simulink model "I_for_2_coils_linear_motion"  (R2021b)
settings: Solver=FixedStepAuto  StartTime=6.4e-3  StopTime=12.76e-3  FixedStep=50e-6  RelTol=1e-3
libraries: simulink x2
(part 1 of 2)
settings Model: Creator=teja  LastModifiedBy=teja

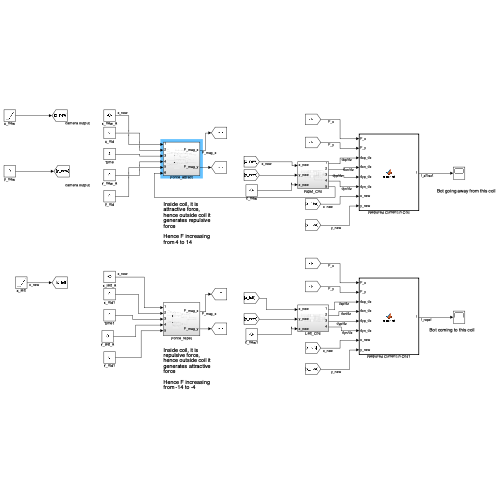
[thumbnail: Simulink's stored preview of the top-level diagram]
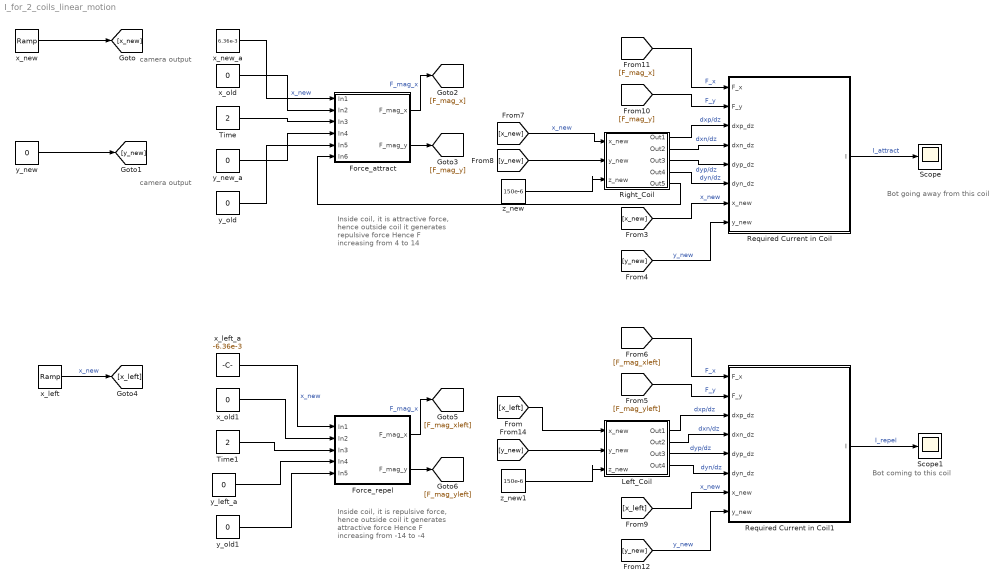
== system I_for_2_coils_linear_motion ==
  note: Bot going away from this coil
  note: Inside coil, it is attractive force, hence outside coil it generates repulsive force
      |
      | Hence F increasing from 4 to 14
  note: camera output
  note: camera output
  note: Inside coil, it is repulsive force, hence outside coil it generates attractive force
      |
      | Hence F increasing from -14 to -4
  note: Bot coming to this coil
  Force_attract : Subsystem
  Force_repel : Subsystem
  Left_Coil : Subsystem
  Required Current in Coil : MATLAB Function  TreatAsAtomicUnit=on
  Required Current in Coil1 : MATLAB Function  TreatAsAtomicUnit=on
  Right_Coil : Subsystem
  Scope : Scope
  Scope1 : Scope
  Time : Constant  Value=2
  Time1 : Constant  Value=2
  x_left : simulink/Sources/Ramp  slope=1  start=0  InitialOutput=-12.76e-3-6.4e-3
  x_left_a : Constant  Value=-6.36e-3
  x_new : simulink/Sources/Ramp  slope=1  start=0  InitialOutput=0
  x_new_a : Constant  Value=6.36e-3
  x_old : Constant  Value=0
  x_old1 : Constant  Value=0
  y_left_a : Constant  Value=0
  y_new : Constant  Value=0
  y_new_a : Constant  Value=0
  y_old : Constant  Value=0
  y_old1 : Constant  Value=0
  z_new : Constant  Value=150e-6
  z_new1 : Constant  Value=150e-6
  wires:
  x_old/1 -> Force_attract/2(In2)
  Time/1 -> Force_attract/3(In3)
  y_old/1 -> Force_attract/5(In5)
  x_new_a/1 -> Force_attract/1(In1)  "x_new"
  y_new/1 -> [y_new]
  y_new_a/1 -> Force_attract/4(In4)
  Force_attract/1(F_mag_x) -> [F_mag_x]  "F_mag_x"
  Force_attract/2(F_mag_y) -> [F_mag_y]
  [F_mag_x] -> Required Current in Coil/1(F_x)  "F_x"
  [F_mag_y] -> Required Current in Coil/2(F_y)  "F_y"
  [x_new] -> Right_Coil/1(x_new)  "x_new"
  [y_new] -> Right_Coil/2(y_new)
  z_new/1 -> Right_Coil/3(z_new)
  Right_Coil/1(Out1) -> Required Current in Coil/3(dxp_dz)  "dxp/dz"
  Right_Coil/2(Out2) -> Required Current in Coil/4(dxn_dz)  "dxn/dz"
  Right_Coil/3(Out3) -> Required Current in Coil/5(dyp_dz)  "dyp/dz"
  Right_Coil/4(Out4) -> Required Current in Coil/6(dyn_dz)  "dyn/dz"
  Required Current in Coil/1(I) -> Scope/1  "I_attract"
  [x_new] -> Required Current in Coil/7(x_new)  "x_new"
  [y_new] -> Required Current in Coil/8(y_new)  "y_new"
  [y_new] -> Required Current in Coil1/8(y_new)  "y_new"
  [x_left] -> Required Current in Coil1/7(x_new)  "x_new"
  Required Current in Coil1/1(I) -> Scope1/1  "I_repel"
  Left_Coil/4(Out4) -> Required Current in Coil1/6(dyn_dz)  "dyn/dz"
  Left_Coil/3(Out3) -> Required Current in Coil1/5(dyp_dz)  "dyp/dz"
  Left_Coil/2(Out2) -> Required Current in Coil1/4(dxn_dz)  "dxn/dz"
  Left_Coil/1(Out1) -> Required Current in Coil1/3(dxp_dz)  "dxp/dz"
  z_new1/1 -> Left_Coil/3(z_new)
  [y_new] -> Left_Coil/2(y_new)
  x_left/1 -> [x_left]  "x_new"
  [F_mag_yleft] -> Required Current in Coil1/2(F_y)  "F_y"
  [F_mag_xleft] -> Required Current in Coil1/1(F_x)  "F_x"
  x_new/1 -> [x_new]
  [x_left] -> Left_Coil/1(x_new)
  Force_repel/2(F_mag_y) -> [F_mag_yleft]
  Force_repel/1(F_mag_x) -> [F_mag_xleft]  "F_mag_x"
  y_left_a/1 -> Force_repel/4(In4)
  x_left_a/1 -> Force_repel/1(In1)  "x_new"
  y_old1/1 -> Force_repel/5(In5)
  Time1/1 -> Force_repel/3(In3)
  x_old1/1 -> Force_repel/2(In2)
  Right_Coil/5(Out5) -> Force_attract/6(In6)

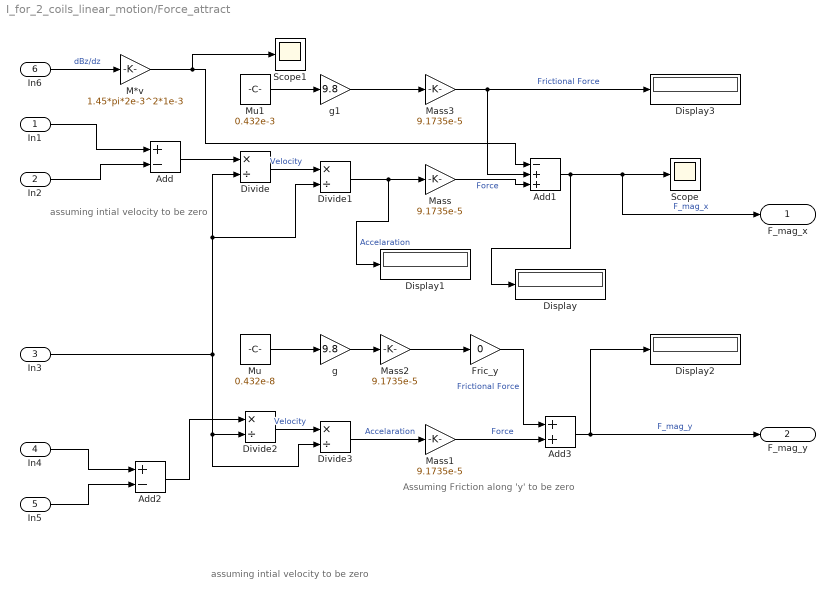
== system I_for_2_coils_linear_motion/Force_attract ==
  note: Assuming Friction along 'y' to be zero
  note: assuming intial velocity to be zero
  note: assuming intial velocity to be zero
  In1 : Inport
  In2 : Inport  Port=2
  In3 : Inport  Port=3
  In4 : Inport  Port=4
  In5 : Inport  Port=5
  In6 : Inport  Port=6
  Add : Sum  Inputs=+-
  Add1 : Sum  Inputs=-++
  Add2 : Sum  Inputs=+-
  Add3 : Sum
  Display{,1..3} (4 alike) : Display
  Divide{,1..3} (4 alike) : Product  Inputs=*/
  Fric_y : Gain  Gain=0
  M*v : Gain  Gain=1.45*pi*2e-3^2*1e-3
  Mass{,1..3} (4 alike) : Gain  Gain=9.1735e-5
  Mu : Constant  Value=0.432e-8
  Mu1 : Constant  Value=0.432e-3
  Scope : Scope
  Scope1 : Scope
  g : Gain  Gain=9.8
  g1 : Gain  Gain=9.8
  F_mag_x : Outport
  F_mag_y : Outport  Port=2
  wires:
  In4/1 -> Add2/1
  Add3/1 -> Display2/1, F_mag_y/1  "F_mag_y"
  In5/1 -> Add2/2
  Mass/1 -> Add1/3  "Force"
  Add2/1 -> Divide2/1
  Mass1/1 -> Add3/2  "Force"
  In1/1 -> Add/1
  Divide/1 -> Divide1/1  "Velocity"
  Add/1 -> Divide/1
  Divide2/1 -> Divide3/1  "Velocity"
  Divide3/1 -> Mass1/1  "Accelaration"
  Divide1/1 -> Display1/1, Mass/1  "Accelaration"
  In3/1 -> Divide/2, Divide1/2, Divide3/2, Divide2/2
  In2/1 -> Add/2
  Add1/1 -> Display/1, F_mag_x/1, Scope/1  "F_mag_x"
  Mu/1 -> g/1
  g/1 -> Mass2/1
  Mass3/1 -> Display3/1, Add1/2  "Frictional Force"
  g1/1 -> Mass3/1
  Mu1/1 -> g1/1
  Mass2/1 -> Fric_y/1
  Fric_y/1 -> Add3/1  "Frictional Force"
  In6/1 -> M*v/1  "dBz/dz"
  M*v/1 -> Scope1/1, Add1/1

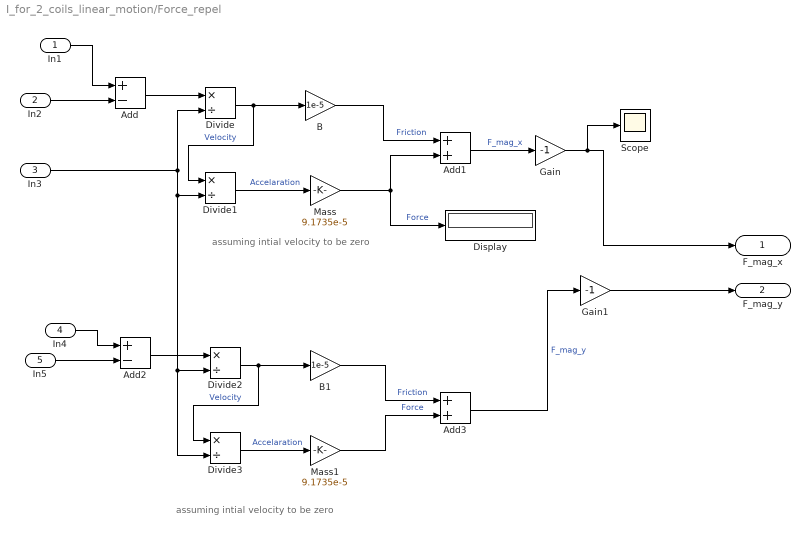
== system I_for_2_coils_linear_motion/Force_repel ==
  note: assuming intial velocity to be zero
  note: assuming intial velocity to be zero
  In1 : Inport
  In2 : Inport  Port=2
  In3 : Inport  Port=3
  In4 : Inport  Port=4
  In5 : Inport  Port=5
  Add : Sum  Inputs=+-
  Add1 : Sum
  Add2 : Sum  Inputs=+-
  Add3 : Sum
  B : Gain  Gain=1e-5
  B1 : Gain  Gain=1e-5
  Display : Display
  Divide{,1..3} (4 alike) : Product  Inputs=*/
  Gain : Gain  Gain=-1
  Gain1 : Gain  Gain=-1
  Mass : Gain  Gain=9.1735e-5
  Mass1 : Gain  Gain=9.1735e-5
  Scope : Scope
  F_mag_x : Outport
  F_mag_y : Outport  Port=2
  wires:
  Add1/1 -> Gain/1  "F_mag_x"
  In2/1 -> Add/2
  In3/1 -> Divide/2, Divide1/2, Divide2/2, Divide3/2
  Divide1/1 -> Mass/1  "Accelaration"
  Divide3/1 -> Mass1/1  "Accelaration"
  Divide2/1 -> Divide3/1, B1/1  "Velocity"
  Add/1 -> Divide/1
  Divide/1 -> B/1, Divide1/1  "Velocity"
  In1/1 -> Add/1
  B/1 -> Add1/1  "Friction"
  Mass1/1 -> Add3/2  "Force"
  B1/1 -> Add3/1  "Friction"
  Add2/1 -> Divide2/1
  Mass/1 -> Add1/2, Display/1  "Force"
  In5/1 -> Add2/2
  Add3/1 -> Gain1/1  "F_mag_y"
  In4/1 -> Add2/1
  Gain/1 -> F_mag_x/1, Scope/1
  Gain1/1 -> F_mag_y/1

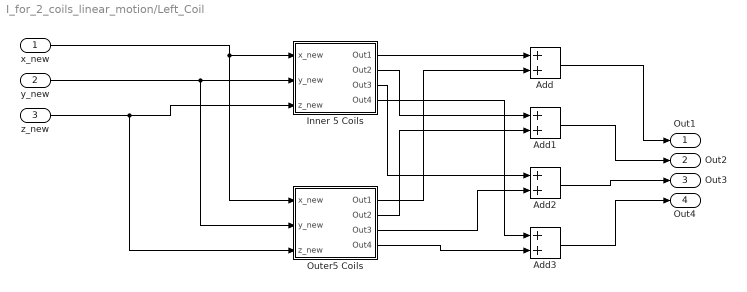
== system I_for_2_coils_linear_motion/Left_Coil ==
  x_new : Inport
  y_new : Inport  Port=2
  z_new : Inport  Port=3
  Add{,1..3} (4 alike) : Sum
  Inner 5 Coils : Subsystem
  Outer5 Coils : Subsystem
  Out1 : Outport
  Out2 : Outport  Port=2
  Out3 : Outport  Port=3
  Out4 : Outport  Port=4
  wires:
  z_new/1 -> Inner 5 Coils/3(z_new), Outer5 Coils/3(z_new)
  Outer5 Coils/4(Out4) -> Add3/2
  Outer5 Coils/1(Out1) -> Add/2
  y_new/1 -> Inner 5 Coils/2(y_new), Outer5 Coils/2(y_new)
  Inner 5 Coils/1(Out1) -> Add/1
  Inner 5 Coils/2(Out2) -> Add1/1
  x_new/1 -> Inner 5 Coils/1(x_new), Outer5 Coils/1(x_new)
  Inner 5 Coils/4(Out4) -> Add3/1
  Add3/1 -> Out4/1
  Inner 5 Coils/3(Out3) -> Add2/1
  Add/1 -> Out1/1
  Outer5 Coils/3(Out3) -> Add2/2
  Outer5 Coils/2(Out2) -> Add1/2
  Add1/1 -> Out2/1
  Add2/1 -> Out3/1

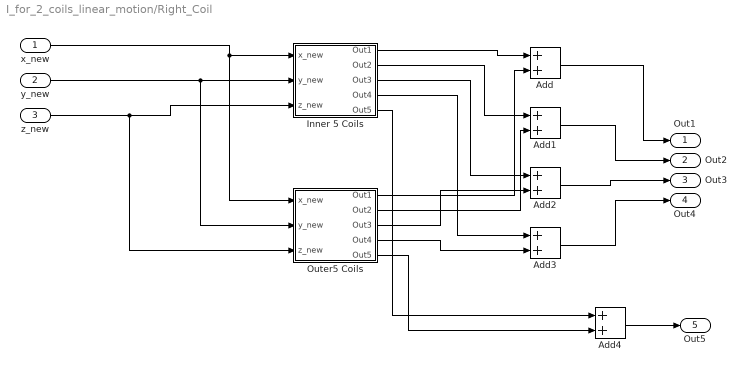
== system I_for_2_coils_linear_motion/Right_Coil ==
  x_new : Inport
  y_new : Inport  Port=2
  z_new : Inport  Port=3
  Add{,1..4} (5 alike) : Sum
  Inner 5 Coils : Subsystem
  Outer5 Coils : Subsystem
  Out1 : Outport
  Out2 : Outport  Port=2
  Out3 : Outport  Port=3
  Out4 : Outport  Port=4
  Out5 : Outport  Port=5
  wires:
  Add2/1 -> Out3/1
  Add1/1 -> Out2/1
  Outer5 Coils/2(Out2) -> Add1/2
  Outer5 Coils/3(Out3) -> Add2/2
  Add/1 -> Out1/1
  Inner 5 Coils/3(Out3) -> Add2/1
  Add3/1 -> Out4/1
  Inner 5 Coils/4(Out4) -> Add3/1
  x_new/1 -> Outer5 Coils/1(x_new), Inner 5 Coils/1(x_new)
  Inner 5 Coils/2(Out2) -> Add1/1
  Inner 5 Coils/1(Out1) -> Add/1
  y_new/1 -> Outer5 Coils/2(y_new), Inner 5 Coils/2(y_new)
  Outer5 Coils/1(Out1) -> Add/2
  Outer5 Coils/4(Out4) -> Add3/2
  z_new/1 -> Outer5 Coils/3(z_new), Inner 5 Coils/3(z_new)
  Outer5 Coils/5(Out5) -> Add4/2
  Inner 5 Coils/5(Out5) -> Add4/1
  Add4/1 -> Out5/1

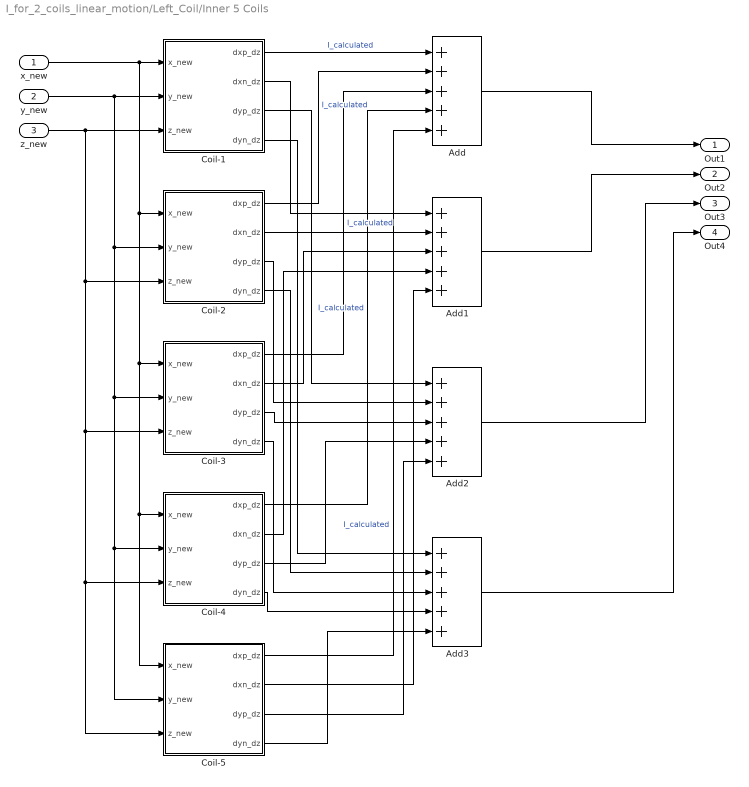
== system I_for_2_coils_linear_motion/Left_Coil/Inner 5 Coils ==
  x_new : Inport
  y_new : Inport  Port=2
  z_new : Inport  Port=3
  Add{,1..3} (4 alike) : Sum  Inputs=+++++
  Coil-1 : MATLAB Function  TreatAsAtomicUnit=on
  Coil-2 : MATLAB Function  TreatAsAtomicUnit=on
  Coil-3 : MATLAB Function  TreatAsAtomicUnit=on
  Coil-4 : MATLAB Function  TreatAsAtomicUnit=on
  Coil-5 : MATLAB Function  TreatAsAtomicUnit=on
  Out1 : Outport
  Out2 : Outport  Port=2
  Out3 : Outport  Port=3
  Out4 : Outport  Port=4
  wires:
  Coil-5/2(dxn_dz) -> Add1/5
  Coil-3/3(dyp_dz) -> Add2/3
  Coil-3/2(dxn_dz) -> Add1/3
  Coil-4/2(dxn_dz) -> Add1/4
  Coil-5/4(dyn_dz) -> Add3/5
  Coil-4/3(dyp_dz) -> Add2/4
  Coil-5/3(dyp_dz) -> Add2/5
  Coil-2/3(dyp_dz) -> Add2/2
  Coil-1/1(dxp_dz) -> Add/1  "I_calculated"
  x_new/1 -> Coil-1/1(x_new), Coil-2/1(x_new), Coil-3/1(x_new), Coil-4/1(x_new), Coil-5/1(x_new)
  Coil-5/1(dxp_dz) -> Add/5  "I_calculated"
  y_new/1 -> Coil-1/2(y_new), Coil-2/2(y_new), Coil-3/2(y_new), Coil-4/2(y_new), Coil-5/2(y_new)
  Coil-1/4(dyn_dz) -> Add3/1
  Coil-4/4(dyn_dz) -> Add3/4
  Coil-1/2(dxn_dz) -> Add1/1
  Coil-1/3(dyp_dz) -> Add2/1
  Coil-2/1(dxp_dz) -> Add/2  "I_calculated"
  Add/1 -> Out1/1
  Coil-4/1(dxp_dz) -> Add/4  "I_calculated"
  z_new/1 -> Coil-2/3(z_new), Coil-5/3(z_new), Coil-4/3(z_new), Coil-3/3(z_new), Coil-1/3(z_new)
  Coil-3/4(dyn_dz) -> Add3/3
  Coil-3/1(dxp_dz) -> Add/3  "I_calculated"
  Add3/1 -> Out4/1
  Coil-2/4(dyn_dz) -> Add3/2
  Coil-2/2(dxn_dz) -> Add1/2
  Add1/1 -> Out2/1
  Add2/1 -> Out3/1

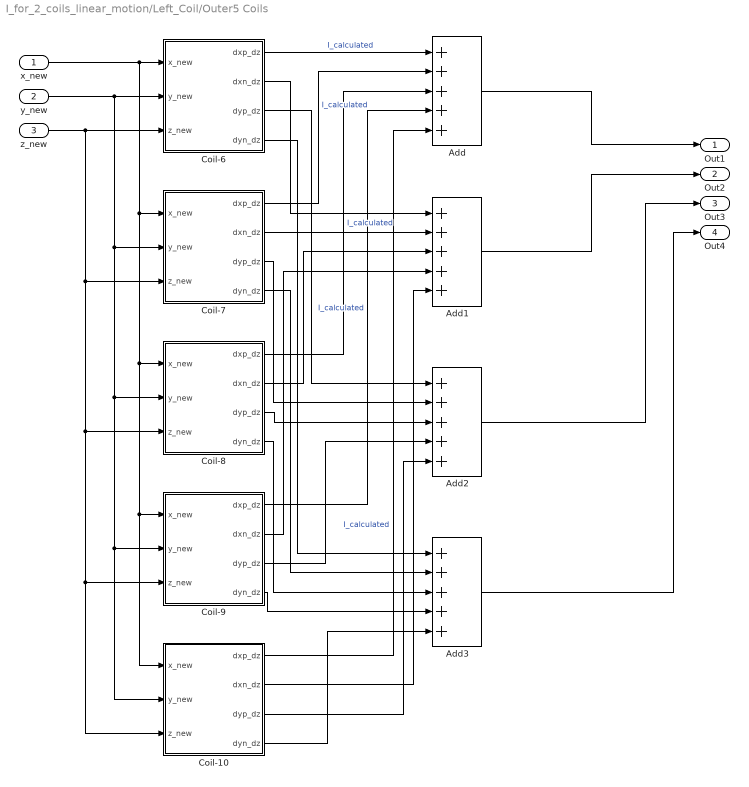
== system I_for_2_coils_linear_motion/Left_Coil/Outer5 Coils ==
  x_new : Inport
  y_new : Inport  Port=2
  z_new : Inport  Port=3
  Add{,1..3} (4 alike) : Sum  Inputs=+++++
  Coil-10 : MATLAB Function  TreatAsAtomicUnit=on
  Coil-6 : MATLAB Function  TreatAsAtomicUnit=on
  Coil-7 : MATLAB Function  TreatAsAtomicUnit=on
  Coil-8 : MATLAB Function  TreatAsAtomicUnit=on
  Coil-9 : MATLAB Function  TreatAsAtomicUnit=on
  Out1 : Outport
  Out2 : Outport  Port=2
  Out3 : Outport  Port=3
  Out4 : Outport  Port=4
  wires:
  Add2/1 -> Out3/1
  Add1/1 -> Out2/1
  Coil-7/2(dxn_dz) -> Add1/2
  Coil-7/4(dyn_dz) -> Add3/2
  Add3/1 -> Out4/1
  Coil-8/1(dxp_dz) -> Add/3  "I_calculated"
  Coil-8/4(dyn_dz) -> Add3/3
  z_new/1 -> Coil-6/3(z_new), Coil-8/3(z_new), Coil-10/3(z_new), Coil-9/3(z_new), Coil-7/3(z_new)
  Coil-9/1(dxp_dz) -> Add/4  "I_calculated"
  Add/1 -> Out1/1
  Coil-7/1(dxp_dz) -> Add/2  "I_calculated"
  Coil-6/3(dyp_dz) -> Add2/1
  Coil-6/2(dxn_dz) -> Add1/1
  Coil-9/4(dyn_dz) -> Add3/4
  Coil-6/4(dyn_dz) -> Add3/1
  y_new/1 -> Coil-10/2(y_new), Coil-9/2(y_new), Coil-8/2(y_new), Coil-7/2(y_new), Coil-6/2(y_new)
  Coil-10/1(dxp_dz) -> Add/5  "I_calculated"
  x_new/1 -> Coil-10/1(x_new), Coil-9/1(x_new), Coil-8/1(x_new), Coil-7/1(x_new), Coil-6/1(x_new)
  Coil-6/1(dxp_dz) -> Add/1  "I_calculated"
  Coil-7/3(dyp_dz) -> Add2/2
  Coil-10/3(dyp_dz) -> Add2/5
  Coil-9/3(dyp_dz) -> Add2/4
  Coil-10/4(dyn_dz) -> Add3/5
  Coil-9/2(dxn_dz) -> Add1/4
  Coil-8/2(dxn_dz) -> Add1/3
  Coil-8/3(dyp_dz) -> Add2/3
  Coil-10/2(dxn_dz) -> Add1/5

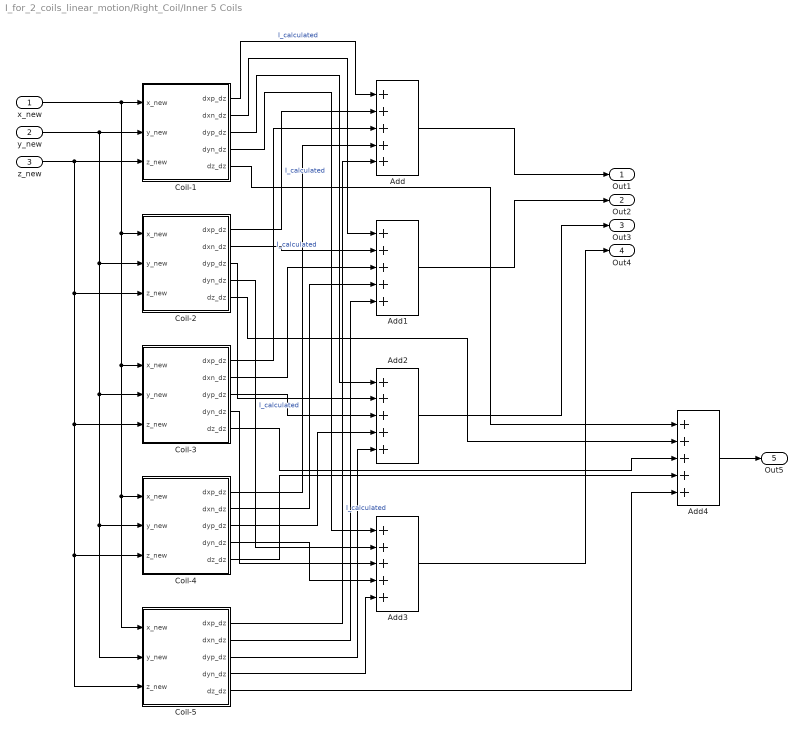
== system I_for_2_coils_linear_motion/Right_Coil/Inner 5 Coils ==
  x_new : Inport
  y_new : Inport  Port=2
  z_new : Inport  Port=3
  Add{,1..4} (5 alike) : Sum  Inputs=+++++
  Coil-1 : MATLAB Function  TreatAsAtomicUnit=on
  Coil-2 : MATLAB Function  TreatAsAtomicUnit=on
  Coil-3 : MATLAB Function  TreatAsAtomicUnit=on
  Coil-4 : MATLAB Function  TreatAsAtomicUnit=on
  Coil-5 : MATLAB Function  TreatAsAtomicUnit=on
  Out1 : Outport
  Out2 : Outport  Port=2
  Out3 : Outport  Port=3
  Out4 : Outport  Port=4
  Out5 : Outport  Port=5
  wires:
  Add2/1 -> Out3/1
  Add1/1 -> Out2/1
  Coil-2/2(dxn_dz) -> Add1/2
  Coil-2/4(dyn_dz) -> Add3/2
  Add3/1 -> Out4/1
  Coil-3/1(dxp_dz) -> Add/3  "I_calculated"
  Coil-3/4(dyn_dz) -> Add3/3
  z_new/1 -> Coil-1/3(z_new), Coil-3/3(z_new), Coil-4/3(z_new), Coil-5/3(z_new), Coil-2/3(z_new)
  Coil-4/1(dxp_dz) -> Add/4  "I_calculated"
  Add/1 -> Out1/1
  Coil-2/1(dxp_dz) -> Add/2  "I_calculated"
  Coil-1/3(dyp_dz) -> Add2/1
  Coil-1/2(dxn_dz) -> Add1/1
  Coil-4/4(dyn_dz) -> Add3/4
  Coil-1/4(dyn_dz) -> Add3/1
  y_new/1 -> Coil-5/2(y_new), Coil-4/2(y_new), Coil-3/2(y_new), Coil-2/2(y_new), Coil-1/2(y_new)
  Coil-5/1(dxp_dz) -> Add/5  "I_calculated"
  x_new/1 -> Coil-5/1(x_new), Coil-4/1(x_new), Coil-3/1(x_new), Coil-2/1(x_new), Coil-1/1(x_new)
  Coil-1/1(dxp_dz) -> Add/1  "I_calculated"
  Coil-2/3(dyp_dz) -> Add2/2
  Coil-5/3(dyp_dz) -> Add2/5
  Coil-4/3(dyp_dz) -> Add2/4
  Coil-5/4(dyn_dz) -> Add3/5
  Coil-4/2(dxn_dz) -> Add1/4
  Coil-3/2(dxn_dz) -> Add1/3
  Coil-3/3(dyp_dz) -> Add2/3
  Coil-5/2(dxn_dz) -> Add1/5
  Coil-1/5(dz_dz) -> Add4/1
  Coil-2/5(dz_dz) -> Add4/2
  Coil-3/5(dz_dz) -> Add4/3
  Coil-4/5(dz_dz) -> Add4/4
  Coil-5/5(dz_dz) -> Add4/5
  Add4/1 -> Out5/1

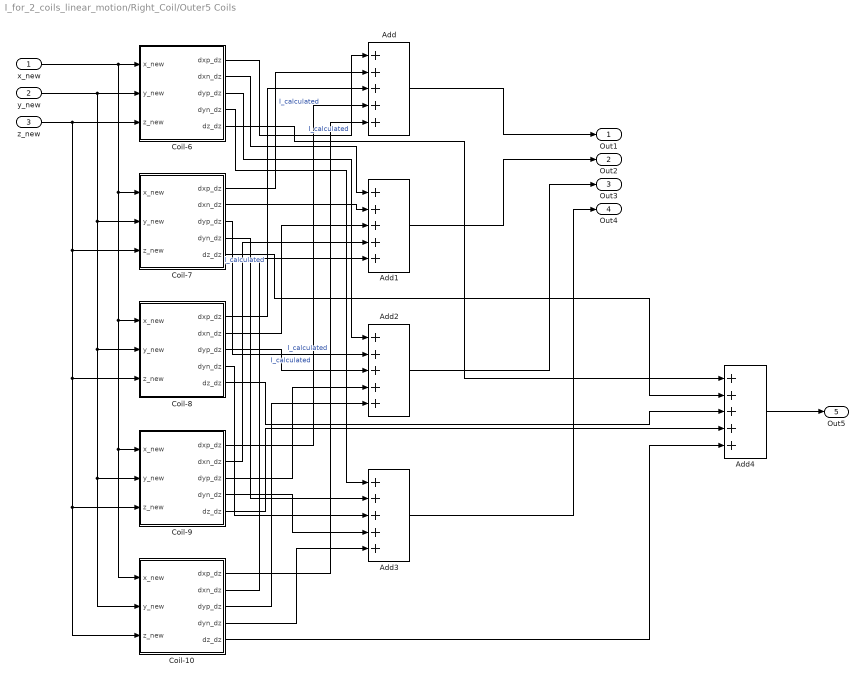
== system I_for_2_coils_linear_motion/Right_Coil/Outer5 Coils ==
  x_new : Inport
  y_new : Inport  Port=2
  z_new : Inport  Port=3
  Add{,1..4} (5 alike) : Sum  Inputs=+++++
  Coil-10 : MATLAB Function  TreatAsAtomicUnit=on
  Coil-6 : MATLAB Function  TreatAsAtomicUnit=on
  Coil-7 : MATLAB Function  TreatAsAtomicUnit=on
  Coil-8 : MATLAB Function  TreatAsAtomicUnit=on
  Coil-9 : MATLAB Function  TreatAsAtomicUnit=on
  Out1 : Outport
  Out2 : Outport  Port=2
  Out3 : Outport  Port=3
  Out4 : Outport  Port=4
  Out5 : Outport  Port=5
  wires:
  Coil-10/2(dxn_dz) -> Add1/5
  Coil-8/3(dyp_dz) -> Add2/3
  Coil-8/2(dxn_dz) -> Add1/3
  Coil-9/2(dxn_dz) -> Add1/4
  Coil-10/4(dyn_dz) -> Add3/5
  Coil-9/3(dyp_dz) -> Add2/4
  Coil-10/3(dyp_dz) -> Add2/5
  Coil-7/3(dyp_dz) -> Add2/2
  Coil-6/1(dxp_dz) -> Add/1  "I_calculated"
  x_new/1 -> Coil-6/1(x_new), Coil-7/1(x_new), Coil-8/1(x_new), Coil-9/1(x_new), Coil-10/1(x_new)
  Coil-10/1(dxp_dz) -> Add/5  "I_calculated"
  y_new/1 -> Coil-6/2(y_new), Coil-7/2(y_new), Coil-8/2(y_new), Coil-9/2(y_new), Coil-10/2(y_new)
  Coil-6/4(dyn_dz) -> Add3/1
  Coil-9/4(dyn_dz) -> Add3/4
  Coil-6/2(dxn_dz) -> Add1/1
  Coil-6/3(dyp_dz) -> Add2/1
  Coil-7/1(dxp_dz) -> Add/2  "I_calculated"
  Add/1 -> Out1/1
  Coil-9/1(dxp_dz) -> Add/4  "I_calculated"
  z_new/1 -> Coil-7/3(z_new), Coil-9/3(z_new), Coil-10/3(z_new), Coil-8/3(z_new), Coil-6/3(z_new)
  Coil-8/4(dyn_dz) -> Add3/3
  Coil-8/1(dxp_dz) -> Add/3  "I_calculated"
  Add3/1 -> Out4/1
  Coil-7/4(dyn_dz) -> Add3/2
  Coil-7/2(dxn_dz) -> Add1/2
  Add1/1 -> Out2/1
  Add2/1 -> Out3/1
  Coil-6/5(dz_dz) -> Add4/1
  Coil-7/5(dz_dz) -> Add4/2
  Coil-8/5(dz_dz) -> Add4/3
  Coil-9/5(dz_dz) -> Add4/4
  Coil-10/5(dz_dz) -> Add4/5
  Add4/1 -> Out5/1

== matlab function I_for_2_coils_linear_motion/Required Current in Coil ==
  data: F_x input; F_y input; I output; dxp_dz input; dxn_dz input; dyp_dz input; dyn_dz input; x_new input; y_new input
function  I = current(F_x, F_y,dxp_dz, dxn_dz, dyp_dz, dyn_dz, x_new, y_new)
radius = 3e-3;%m
height = 1e-3;%m
Magentization = 1.45; %T
m0 = 4*pi*10e-7;
vol_cy = pi*radius^2*height; % If Object is Cylinder, vol in m^3
if F_y == 0 && x_new ~= 0
        I = (F_x/ (dxp_dz + dxn_dz))* m0/ (vol_cy * Magentization);
    elseif F_x == 0 && y_new ~= 0
        I = (F_y / (dyp_dz + dyn_dz))* m0/ (vol_cy * Magentization);
    elseif F_x== 0 && F_y == 0 
        I = 0;
    else
        I = (F_x/ (dxp_dz + dxn_dz)+  F_y / (dyp_dz + dyn_dz))* m0/ (vol_cy * Magentization);
end
end

== matlab function I_for_2_coils_linear_motion/Right_Coil/Outer5 Coils/Coil-6 ==
  data: dxp_dz output; x_new input; y_new input; z_new input; dxn_dz output; dyp_dz output; dyn_dz output; dz_dz output
function  [dxp_dz, dxn_dz, dyp_dz, dyn_dz, dz_dz] = current(x_new, y_new, z_new)

g = 420e-6;     %Coil spacing
m0 = 4*pi*1e-7;
radius = 3e-3;%m
height = 1e-3;%m
Magentization = 1.45; %T
vol_cy = pi*radius^2*height; % If Object is Cylinder, vol in m^3
% vol_sp = (4/3)*(pi * radius^3); % If Object is Sphere, vol in m^3

k = 0.4e-3; %additional length added to wires, to get concentric coil
%--------%--------%--------%--------%--------%--------%--------%----------
% Line along y - axis
%-%--------%--------%--------%--------%--------%--------%--------%--------
yp1_1 = -0.6e-3 - 5*k;
yp2_1 = 0.6e-3 + 5*k;
yn1_1 = -0.8e-3 - 5*k;
yn2_1 = 0.8e-3 + 5*k;
a_xp_1 = 6*g;  
a_xn_1 = -6*g;

k_yp_1 = 1/(4*pi*((a_xp_1-x_new)^2+z_new^2));
k_1yp_1 = (yp2_1-y_new)/((yp2_1-y_new)^2+(a_xp_1-x_new)^2+z_new^2)^0.5;
k_2yp_1 = (yp1_1-y_new)/((yp1_1-y_new)^2+(a_xp_1-x_new)^2+z_new^2)^0.5;

k_1yp_3 = (yp2_1-y_new)/((yp2_1-y_new)^2+(a_xp_1-x_new)^2+z_new^2)^1.5;
k_2yp_3 = (yp1_1-y_new)/((yp1_1-y_new)^2+(a_xp_1-x_new)^2+z_new^2)^1.5;

k_yn_1 = 1/(4*pi*((a_xn_1-x_new)^2+z_new^2));
k_1yn_1 = (yn2_1-y_new)/((yn2_1-y_new)^2+(a_xn_1-x_new)^2+z_new^2)^0.5;
k_2yn_1 = (yn1_1-y_new)/((yn1_1-y_new)^2+(a_xn_1-x_new)^2+z_new^2)^0.5;

k_1yn_3 = (yn2_1-y_new)/((yn2_1-y_new)^2+(a_xn_1-x_new)^2+z_new^2)^1.5;
k_2yn_3 = (yn1_1-y_new)/((yn1_1-y_new)^2+(a_xn_1-x_new)^2+z_new^2)^1.5;


hyp_z_1 = (k_yp_1) *m0;
hyp_z1_1 = (k_1yp_1 - k_2yp_1)*(-1);
hyp_z2_1 = (k_yp_1*(k_1yp_1 - k_2yp_1)*(z_new^2))*4*pi*2;
hyp_z3_1 = (k_1yp_3 - k_2yp_3)*(z_new^2);
dxp_dz = hyp_z_1*(hyp_z1_1 + hyp_z2_1 + hyp_z3_1);


hyn_z_1 = (k_yn_1)* m0*(-1);
hyn_z1_1 = (k_1yn_1 - k_2yn_1)*(-1);
hyn_z2_1 = (k_yn_1*(k_1yn_1 - k_2yn_1)*(z_new^2))*4*pi*2;
hyn_z3_1 = (k_1yn_3 - k_2yn_3)*(z_new^2);
dxn_dz = hyn_z_1*(hyn_z1_1 + hyn_z2_1 + hyn_z3_1);

%--------%--------%--------%--------%--------%--------%--------%----------
% Line along x - axis
%-%--------%--------%--------%--------%a--------%--------%--------%--------
xp1_1 = -0.8e-3 - 5*k;
xp2_1 = 0.8e-3 + 5*k;
xn1_1 = -1e-3 - 5*k;
xn2_1 = 1e-3 + 5*k;
a_yp_1 = 2.675;          %Distance of coil from (0,0)
a_yn_1 = -2.675;

k_xp_1 = 1/(4*pi*((a_yp_1-y_new)^2+z_new^2));
k_1xp_1 = (xp2_1-x_new)/((xp2_1-x_new)^2+(a_yp_1-y_new)^2+z_new^2)^0.5;
k_2xp_1 = (xp1_1-x_new)/((xp1_1-x_new)^2+(a_yp_1-y_new)^2+z_new^2)^0.5;

k_xn_1 = 1/(4*pi*((a_yn_1-y_new)^2+z_new^2));
k_1xn_1 = (xn2_1-x_new)/((xn2_1-x_new)^2+(a_yn_1-y_new)^2+z_new^2)^0.5;
k_2xn_1 = (xn1_1-x_new)/((xn1_1-x_new)^2+(a_yn_1-y_new)^2+z_new^2)^0.5;

k_1xp_3 = (xp2_1-x_new)/((xp2_1-x_new)^2+(a_yp_1-y_new)^2+z_new^2)^1.5;
k_2xp_3 = (xp1_1-x_new)/((xp1_1-x_new)^2+(a_yp_1-y_new)^2+z_new^2)^1.5;

k_1xn_3 = (xn2_1-x_new)/((xn2_1-x_new)^2+(a_yn_1-y_new)^2+z_new^2)^1.5;
k_2xn_3 = (xn1_1-x_new)/((xn1_1-x_new)^2+(a_yn_1-y_new)^2+z_new^2)^1.5;


hxp_z_1 = (k_xp_1)*m0;
hxp_z1_1 = (k_1xp_1 - k_2xp_1)*(-1);
hxp_z2_1 = (k_xp_1*(k_1xp_1 - k_2xp_1)*(z_new^2))*4*pi*2;
hxp_z3_1 = (k_1xp_3 - k_2xp_3)*(z_new^2);
dyp_dz = hxp_z_1*(hxp_z1_1 + hxp_z2_1 + hxp_z3_1);


hxn_z_1 = (k_xn_1)*m0*(-1);
hxn_z1_1 = (k_1xn_1 - k_2xn_1)*(-1);
hxn_z2_1 = (k_xn_1*(k_1xn_1 - k_2xn_1)*(z_new^2))*4*pi*2;
hxn_z3_1 = (k_1xn_3 - k_2xn_3)*(z_new^2);
dyn_dz = hxn_z_1*(hxn_z1_1 + hxn_z2_1 + hxn_z3_1);

hzp_z_1 = (k_yp_1) *m0 * ((a_yp_1-y_new)+(a_xp_1-x_new)) * z_new ;
hzp_z1_1 = (k_1yp_1 - k_2yp_1 + k_1xp_1 - k_2xp_1)*(-2);
hzp_z3_1 = (k_1yp_3 - k_2yp_3 + k_1xp_3 - k_2xp_3);
dzp_dz = hzp_z_1*(hzp_z1_1 + hzp_z3_1);

hzn_z_1 = (k_yp_1) *m0 *(-1) * ((a_yn_1-y_new)+(a_xn_1-x_new)) * z_new;
hzn_z1_1 =(k_1yn_1 - k_2yn_1 + k_1xn_1 - k_2xn_1)*(-2);
hzn_z3_1 = (k_1yn_3 - k_2yn_3 + k_1xn_3 - k_2xn_3);
dzn_dz = hzn_z_1*(hzn_z1_1 + hzn_z3_1);

dz_dz = dzp_dz + dzn_dz;

end

== matlab function I_for_2_coils_linear_motion/Right_Coil/Outer5 Coils/Coil-7 ==
  data: dxp_dz output; x_new input; y_new input; z_new input; dxn_dz output; dyp_dz output; dyn_dz output; dz_dz output
function  [dxp_dz, dxn_dz, dyp_dz, dyn_dz, dz_dz] = current(x_new, y_new, z_new)

g = 417.14e-6;     %Coil spacing
m0 = 4*pi*1e-7;
radius = 3e-3;%m
height = 1e-3;%m
Magentization = 1.45; %T
vol_cy = pi*radius^2*height; % If Object is Cylinder, vol in m^3
% vol_sp = (4/3)*(pi * radius^3); % If Object is Sphere, vol in m^3

k = 0.4e-3; %additional length added to wires, to get concentric coil
%--------%--------%--------%--------%--------%--------%--------%----------
% Line along y - axis
%-%--------%--------%--------%--------%--------%--------%--------%--------
yp1_1 = -0.6e-3 - 6*k;
yp2_1 = 0.6e-3 + 6*k;
yn1_1 = -0.8e-3 - 6*k;
yn2_1 = 0.8e-3 + 6*k;
a_xp_1 = 7*g;  
a_xn_1 = -7*g;

k_yp_1 = 1/(4*pi*((a_xp_1-x_new)^2+z_new^2));
k_1yp_1 = (yp2_1-y_new)/((yp2_1-y_new)^2+(a_xp_1-x_new)^2+z_new^2)^0.5;
k_2yp_1 = (yp1_1-y_new)/((yp1_1-y_new)^2+(a_xp_1-x_new)^2+z_new^2)^0.5;

k_1yp_3 = (yp2_1-y_new)/((yp2_1-y_new)^2+(a_xp_1-x_new)^2+z_new^2)^1.5;
k_2yp_3 = (yp1_1-y_new)/((yp1_1-y_new)^2+(a_xp_1-x_new)^2+z_new^2)^1.5;

k_yn_1 = 1/(4*pi*((a_xn_1-x_new)^2+z_new^2));
k_1yn_1 = (yn2_1-y_new)/((yn2_1-y_new)^2+(a_xn_1-x_new)^2+z_new^2)^0.5;
k_2yn_1 = (yn1_1-y_new)/((yn1_1-y_new)^2+(a_xn_1-x_new)^2+z_new^2)^0.5;

k_1yn_3 = (yn2_1-y_new)/((yn2_1-y_new)^2+(a_xn_1-x_new)^2+z_new^2)^1.5;
k_2yn_3 = (yn1_1-y_new)/((yn1_1-y_new)^2+(a_xn_1-x_new)^2+z_new^2)^1.5;


hyp_z_1 = (k_yp_1) *m0;
hyp_z1_1 = (k_1yp_1 - k_2yp_1)*(-1);
hyp_z2_1 = (k_yp_1*(k_1yp_1 - k_2yp_1)*(z_new^2))*4*pi*2;
hyp_z3_1 = (k_1yp_3 - k_2yp_3)*(z_new^2);
dxp_dz = hyp_z_1*(hyp_z1_1 + hyp_z2_1 + hyp_z3_1);


hyn_z_1 = (k_yn_1)* m0*(-1);
hyn_z1_1 = (k_1yn_1 - k_2yn_1)*(-1);
hyn_z2_1 = (k_yn_1*(k_1yn_1 - k_2yn_1)*(z_new^2))*4*pi*2;
hyn_z3_1 = (k_1yn_3 - k_2yn_3)*(z_new^2);
dxn_dz = hyn_z_1*(hyn_z1_1 + hyn_z2_1 + hyn_z3_1);

%--------%--------%--------%--------%--------%--------%--------%----------
% Line along x - axis
%-%--------%--------%--------%--------%a--------%--------%--------%--------
xp1_1 = -0.8e-3 - 6*k;
xp2_1 = 0.8e-3 + 6*k;
xn1_1 = -1e-3 - 6*k;
xn2_1 = 1e-3 + 6*k;
a_yp_1 = 3.075;          %Distance of coil from (0,0)
a_yn_1 = -3.075;

k_xp_1 = 1/(4*pi*((a_yp_1-y_new)^2+z_new^2));
k_1xp_1 = (xp2_1-x_new)/((xp2_1-x_new)^2+(a_yp_1-y_new)^2+z_new^2)^0.5;
k_2xp_1 = (xp1_1-x_new)/((xp1_1-x_new)^2+(a_yp_1-y_new)^2+z_new^2)^0.5;

k_xn_1 = 1/(4*pi*((a_yn_1-y_new)^2+z_new^2));
k_1xn_1 = (xn2_1-x_new)/((xn2_1-x_new)^2+(a_yn_1-y_new)^2+z_new^2)^0.5;
k_2xn_1 = (xn1_1-x_new)/((xn1_1-x_new)^2+(a_yn_1-y_new)^2+z_new^2)^0.5;

k_1xp_3 = (xp2_1-x_new)/((xp2_1-x_new)^2+(a_yp_1-y_new)^2+z_new^2)^1.5;
k_2xp_3 = (xp1_1-x_new)/((xp1_1-x_new)^2+(a_yp_1-y_new)^2+z_new^2)^1.5;

k_1xn_3 = (xn2_1-x_new)/((xn2_1-x_new)^2+(a_yn_1-y_new)^2+z_new^2)^1.5;
k_2xn_3 = (xn1_1-x_new)/((xn1_1-x_new)^2+(a_yn_1-y_new)^2+z_new^2)^1.5;


hxp_z_1 = (k_xp_1)*m0;
hxp_z1_1 = (k_1xp_1 - k_2xp_1)*(-1);
hxp_z2_1 = (k_xp_1*(k_1xp_1 - k_2xp_1)*(z_new^2))*4*pi*2;
hxp_z3_1 = (k_1xp_3 - k_2xp_3)*(z_new^2);
dyp_dz = hxp_z_1*(hxp_z1_1 + hxp_z2_1 + hxp_z3_1);


hxn_z_1 = (k_xn_1)*m0*(-1);
hxn_z1_1 = (k_1xn_1 - k_2xn_1)*(-1);
hxn_z2_1 = (k_xn_1*(k_1xn_1 - k_2xn_1)*(z_new^2))*4*pi*2;
hxn_z3_1 = (k_1xn_3 - k_2xn_3)*(z_new^2);
dyn_dz = hxn_z_1*(hxn_z1_1 + hxn_z2_1 + hxn_z3_1);

hzp_z_1 = (k_yp_1) *m0 * ((a_yp_1-y_new)+(a_xp_1-x_new)) * z_new ;
hzp_z1_1 = (k_1yp_1 - k_2yp_1 + k_1xp_1 - k_2xp_1)*(-2);
hzp_z3_1 = (k_1yp_3 - k_2yp_3 + k_1xp_3 - k_2xp_3);
dzp_dz = hzp_z_1*(hzp_z1_1 + hzp_z3_1);

hzn_z_1 = (k_yp_1) *m0 *(-1) * ((a_yn_1-y_new)+(a_xn_1-x_new)) * z_new;
hzn_z1_1 =(k_1yn_1 - k_2yn_1 + k_1xn_1 - k_2xn_1)*(-2);
hzn_z3_1 = (k_1yn_3 - k_2yn_3 + k_1xn_3 - k_2xn_3);
dzn_dz = hzn_z_1*(hzn_z1_1 + hzn_z3_1);

dz_dz = dzp_dz + dzn_dz;

end

== matlab function I_for_2_coils_linear_motion/Right_Coil/Outer5 Coils/Coil-8 ==
  data: dxp_dz output; x_new input; y_new input; z_new input; dxn_dz output; dyp_dz output; dyn_dz output; dz_dz output
function  [dxp_dz, dxn_dz, dyp_dz, dyn_dz, dz_dz] = current(x_new, y_new, z_new)

g = 415e-6;     %Coil spacing
m0 = 4*pi*1e-7;
radius = 3e-3;%m
height = 1e-3;%m
Magentization = 1.45; %T
vol_cy = pi*radius^2*height; % If Object is Cylinder, vol in m^3
% vol_sp = (4/3)*(pi * radius^3); % If Object is Sphere, vol in m^3

k = 0.4e-3; %additional length added to wires, to get concentric coil
%--------%--------%--------%--------%--------%--------%--------%----------
% Line along y - axis
%-%--------%--------%--------%--------%--------%--------%--------%--------
yp1_1 = -0.6e-3 - 7*k;
yp2_1 = 0.6e-3 + 7*k;
yn1_1 = -0.8e-3 - 7*k;
yn2_1 = 0.8e-3 + 7*k;
a_xp_1 = 8*g;  
a_xn_1 = -8*g;

k_yp_1 = 1/(4*pi*((a_xp_1-x_new)^2+z_new^2));
k_1yp_1 = (yp2_1-y_new)/((yp2_1-y_new)^2+(a_xp_1-x_new)^2+z_new^2)^0.5;
k_2yp_1 = (yp1_1-y_new)/((yp1_1-y_new)^2+(a_xp_1-x_new)^2+z_new^2)^0.5;

k_1yp_3 = (yp2_1-y_new)/((yp2_1-y_new)^2+(a_xp_1-x_new)^2+z_new^2)^1.5;
k_2yp_3 = (yp1_1-y_new)/((yp1_1-y_new)^2+(a_xp_1-x_new)^2+z_new^2)^1.5;

k_yn_1 = 1/(4*pi*((a_xn_1-x_new)^2+z_new^2));
k_1yn_1 = (yn2_1-y_new)/((yn2_1-y_new)^2+(a_xn_1-x_new)^2+z_new^2)^0.5;
k_2yn_1 = (yn1_1-y_new)/((yn1_1-y_new)^2+(a_xn_1-x_new)^2+z_new^2)^0.5;

k_1yn_3 = (yn2_1-y_new)/((yn2_1-y_new)^2+(a_xn_1-x_new)^2+z_new^2)^1.5;
k_2yn_3 = (yn1_1-y_new)/((yn1_1-y_new)^2+(a_xn_1-x_new)^2+z_new^2)^1.5;


hyp_z_1 = (k_yp_1) *m0;
hyp_z1_1 = (k_1yp_1 - k_2yp_1)*(-1);
hyp_z2_1 = (k_yp_1*(k_1yp_1 - k_2yp_1)*(z_new^2))*4*pi*2;
hyp_z3_1 = (k_1yp_3 - k_2yp_3)*(z_new^2);
dxp_dz = hyp_z_1*(hyp_z1_1 + hyp_z2_1 + hyp_z3_1);


hyn_z_1 = (k_yn_1)* m0*(-1);
hyn_z1_1 = (k_1yn_1 - k_2yn_1)*(-1);
hyn_z2_1 = (k_yn_1*(k_1yn_1 - k_2yn_1)*(z_new^2))*4*pi*2;
hyn_z3_1 = (k_1yn_3 - k_2yn_3)*(z_new^2);
dxn_dz = hyn_z_1*(hyn_z1_1 + hyn_z2_1 + hyn_z3_1);

%--------%--------%--------%--------%--------%--------%--------%----------
% Line along x - axis
%-%--------%--------%--------%--------%a--------%--------%--------%--------
xp1_1 = -0.8e-3 - 7*k;
xp2_1 = 0.8e-3 + 7*k;
xn1_1 = -1e-3 - 7*k;
xn2_1 = 1e-3 + 7*k;
a_yp_1 = 3.475;          %Distance of coil from (0,0)
a_yn_1 = -3.475;

k_xp_1 = 1/(4*pi*((a_yp_1-y_new)^2+z_new^2));
k_1xp_1 = (xp2_1-x_new)/((xp2_1-x_new)^2+(a_yp_1-y_new)^2+z_new^2)^0.5;
k_2xp_1 = (xp1_1-x_new)/((xp1_1-x_new)^2+(a_yp_1-y_new)^2+z_new^2)^0.5;

k_xn_1 = 1/(4*pi*((a_yn_1-y_new)^2+z_new^2));
k_1xn_1 = (xn2_1-x_new)/((xn2_1-x_new)^2+(a_yn_1-y_new)^2+z_new^2)^0.5;
k_2xn_1 = (xn1_1-x_new)/((xn1_1-x_new)^2+(a_yn_1-y_new)^2+z_new^2)^0.5;

k_1xp_3 = (xp2_1-x_new)/((xp2_1-x_new)^2+(a_yp_1-y_new)^2+z_new^2)^1.5;
k_2xp_3 = (xp1_1-x_new)/((xp1_1-x_new)^2+(a_yp_1-y_new)^2+z_new^2)^1.5;

k_1xn_3 = (xn2_1-x_new)/((xn2_1-x_new)^2+(a_yn_1-y_new)^2+z_new^2)^1.5;
k_2xn_3 = (xn1_1-x_new)/((xn1_1-x_new)^2+(a_yn_1-y_new)^2+z_new^2)^1.5;


hxp_z_1 = (k_xp_1)*m0;
hxp_z1_1 = (k_1xp_1 - k_2xp_1)*(-1);
hxp_z2_1 = (k_xp_1*(k_1xp_1 - k_2xp_1)*(z_new^2))*4*pi*2;
hxp_z3_1 = (k_1xp_3 - k_2xp_3)*(z_new^2);
dyp_dz = hxp_z_1*(hxp_z1_1 + hxp_z2_1 + hxp_z3_1);


hxn_z_1 = (k_xn_1)*m0*(-1);
hxn_z1_1 = (k_1xn_1 - k_2xn_1)*(-1);
hxn_z2_1 = (k_xn_1*(k_1xn_1 - k_2xn_1)*(z_new^2))*4*pi*2;
hxn_z3_1 = (k_1xn_3 - k_2xn_3)*(z_new^2);
dyn_dz = hxn_z_1*(hxn_z1_1 + hxn_z2_1 + hxn_z3_1);

hzp_z_1 = (k_yp_1) *m0 * ((a_yp_1-y_new)+(a_xp_1-x_new)) * z_new ;
hzp_z1_1 = (k_1yp_1 - k_2yp_1 + k_1xp_1 - k_2xp_1)*(-2);
hzp_z3_1 = (k_1yp_3 - k_2yp_3 + k_1xp_3 - k_2xp_3);
dzp_dz = hzp_z_1*(hzp_z1_1 + hzp_z3_1);

hzn_z_1 = (k_yp_1) *m0 *(-1) * ((a_yn_1-y_new)+(a_xn_1-x_new)) * z_new;
hzn_z1_1 =(k_1yn_1 - k_2yn_1 + k_1xn_1 - k_2xn_1)*(-2);
hzn_z3_1 = (k_1yn_3 - k_2yn_3 + k_1xn_3 - k_2xn_3);
dzn_dz = hzn_z_1*(hzn_z1_1 + hzn_z3_1);

dz_dz = dzp_dz + dzn_dz;

end

== matlab function I_for_2_coils_linear_motion/Required Current in Coil1 ==
  data: F_x input; F_y input; I output; dxp_dz input; dxn_dz input; dyp_dz input; dyn_dz input; x_new input; y_new input
function  I = current(F_x, F_y,dxp_dz, dxn_dz, dyp_dz, dyn_dz, x_new, y_new)
radius = 3e-3;%m
height = 1e-3;%m
Magentization = 1.45; %T
m0 = 4*pi*10e-7;
vol_cy = pi*radius^2*height; % If Object is Cylinder, vol in m^3
if F_y == 0 && x_new ~= 0
        I = (F_x/ (dxp_dz + dxn_dz))* m0/ (vol_cy * Magentization);
    elseif F_x == 0 && y_new ~= 0
        I = (F_y / (dyp_dz + dyn_dz))* m0/ (vol_cy * Magentization);
    elseif F_x== 0 && F_y == 0 
        I = 0;
    else
        I = (F_x/ (dxp_dz + dxn_dz)+  F_y / (dyp_dz + dyn_dz))* m0/ (vol_cy * Magentization);
end
end

== matlab function I_for_2_coils_linear_motion/Right_Coil/Outer5 Coils/Coil-10 ==
  data: dxp_dz output; x_new input; y_new input; z_new input; dxn_dz output; dyp_dz output; dyn_dz output; dz_dz output
function  [dxp_dz, dxn_dz, dyp_dz, dyn_dz, dz_dz] = current(x_new, y_new, z_new)

g = 412e-6;     %Coil spacing
m0 = 4*pi*1e-7;
radius = 3e-3;%m
height = 1e-3;%m
Magentization = 1.45; %T
vol_cy = pi*radius^2*height; % If Object is Cylinder, vol in m^3
% vol_sp = (4/3)*(pi * radius^3); % If Object is Sphere, vol in m^3

k = 0.4e-3; %additional length added to wires, to get concentric coil
%--------%--------%--------%--------%--------%--------%--------%----------
% Line along y - axis
%-%--------%--------%--------%--------%--------%--------%--------%--------
yp1_1 = -0.6e-3 - 9*k;
yp2_1 = 0.6e-3 + 9*k;
yn1_1 = -0.8e-3 - 9*k;
yn2_1 = 0.8e-3 + 9*k;
a_xp_1 = 10*g;  
a_xn_1 = -10*g;

k_yp_1 = 1/(4*pi*((a_xp_1-x_new)^2+z_new^2));
k_1yp_1 = (yp2_1-y_new)/((yp2_1-y_new)^2+(a_xp_1-x_new)^2+z_new^2)^0.5;
k_2yp_1 = (yp1_1-y_new)/((yp1_1-y_new)^2+(a_xp_1-x_new)^2+z_new^2)^0.5;

k_1yp_3 = (yp2_1-y_new)/((yp2_1-y_new)^2+(a_xp_1-x_new)^2+z_new^2)^1.5;
k_2yp_3 = (yp1_1-y_new)/((yp1_1-y_new)^2+(a_xp_1-x_new)^2+z_new^2)^1.5;

k_yn_1 = 1/(4*pi*((a_xn_1-x_new)^2+z_new^2));
k_1yn_1 = (yn2_1-y_new)/((yn2_1-y_new)^2+(a_xn_1-x_new)^2+z_new^2)^0.5;
k_2yn_1 = (yn1_1-y_new)/((yn1_1-y_new)^2+(a_xn_1-x_new)^2+z_new^2)^0.5;

k_1yn_3 = (yn2_1-y_new)/((yn2_1-y_new)^2+(a_xn_1-x_new)^2+z_new^2)^1.5;
k_2yn_3 = (yn1_1-y_new)/((yn1_1-y_new)^2+(a_xn_1-x_new)^2+z_new^2)^1.5;


hyp_z_1 = (k_yp_1) *m0;
hyp_z1_1 = (k_1yp_1 - k_2yp_1)*(-1);
hyp_z2_1 = (k_yp_1*(k_1yp_1 - k_2yp_1)*(z_new^2))*4*pi*2;
hyp_z3_1 = (k_1yp_3 - k_2yp_3)*(z_new^2);
dxp_dz = hyp_z_1*(hyp_z1_1 + hyp_z2_1 + hyp_z3_1);


hyn_z_1 = (k_yn_1)* m0*(-1);
hyn_z1_1 = (k_1yn_1 - k_2yn_1)*(-1);
hyn_z2_1 = (k_yn_1*(k_1yn_1 - k_2yn_1)*(z_new^2))*4*pi*2;
hyn_z3_1 = (k_1yn_3 - k_2yn_3)*(z_new^2);
dxn_dz = hyn_z_1*(hyn_z1_1 + hyn_z2_1 + hyn_z3_1);

%--------%--------%--------%--------%--------%--------%--------%----------
% Line along x - axis
%-%--------%--------%--------%--------%a--------%--------%--------%--------
xp1_1 = -0.8e-3 - 9*k;
xp2_1 = 0.8e-3 + 9*k;
xn1_1 = -1e-3 - 9*k;
xn2_1 = 1e-3 + 9*k;
a_yp_1 = 4.275;          %Distance of coil from (0,0)
a_yn_1 = -4.275;

k_xp_1 = 1/(4*pi*((a_yp_1-y_new)^2+z_new^2));
k_1xp_1 = (xp2_1-x_new)/((xp2_1-x_new)^2+(a_yp_1-y_new)^2+z_new^2)^0.5;
k_2xp_1 = (xp1_1-x_new)/((xp1_1-x_new)^2+(a_yp_1-y_new)^2+z_new^2)^0.5;

k_xn_1 = 1/(4*pi*((a_yn_1-y_new)^2+z_new^2));
k_1xn_1 = (xn2_1-x_new)/((xn2_1-x_new)^2+(a_yn_1-y_new)^2+z_new^2)^0.5;
k_2xn_1 = (xn1_1-x_new)/((xn1_1-x_new)^2+(a_yn_1-y_new)^2+z_new^2)^0.5;

k_1xp_3 = (xp2_1-x_new)/((xp2_1-x_new)^2+(a_yp_1-y_new)^2+z_new^2)^1.5;
k_2xp_3 = (xp1_1-x_new)/((xp1_1-x_new)^2+(a_yp_1-y_new)^2+z_new^2)^1.5;

k_1xn_3 = (xn2_1-x_new)/((xn2_1-x_new)^2+(a_yn_1-y_new)^2+z_new^2)^1.5;
k_2xn_3 = (xn1_1-x_new)/((xn1_1-x_new)^2+(a_yn_1-y_new)^2+z_new^2)^1.5;


hxp_z_1 = (k_xp_1)*m0;
hxp_z1_1 = (k_1xp_1 - k_2xp_1)*(-1);
hxp_z2_1 = (k_xp_1*(k_1xp_1 - k_2xp_1)*(z_new^2))*4*pi*2;
hxp_z3_1 = (k_1xp_3 - k_2xp_3)*(z_new^2);
dyp_dz = hxp_z_1*(hxp_z1_1 + hxp_z2_1 + hxp_z3_1);


hxn_z_1 = (k_xn_1)*m0*(-1);
hxn_z1_1 = (k_1xn_1 - k_2xn_1)*(-1);
hxn_z2_1 = (k_xn_1*(k_1xn_1 - k_2xn_1)*(z_new^2))*4*pi*2;
hxn_z3_1 = (k_1xn_3 - k_2xn_3)*(z_new^2);
dyn_dz = hxn_z_1*(hxn_z1_1 + hxn_z2_1 + hxn_z3_1);

hzp_z_1 = (k_yp_1) *m0 * ((a_yp_1-y_new)+(a_xp_1-x_new)) * z_new ;
hzp_z1_1 = (k_1yp_1 - k_2yp_1 + k_1xp_1 - k_2xp_1)*(-2);
hzp_z3_1 = (k_1yp_3 - k_2yp_3 + k_1xp_3 - k_2xp_3);
dzp_dz = hzp_z_1*(hzp_z1_1 + hzp_z3_1);

hzn_z_1 = (k_yp_1) *m0 *(-1) * ((a_yn_1-y_new)+(a_xn_1-x_new)) * z_new;
hzn_z1_1 =(k_1yn_1 - k_2yn_1 + k_1xn_1 - k_2xn_1)*(-2);
hzn_z3_1 = (k_1yn_3 - k_2yn_3 + k_1xn_3 - k_2xn_3);
dzn_dz = hzn_z_1*(hzn_z1_1 + hzn_z3_1);

dz_dz = dzp_dz + dzn_dz;

end

== matlab function I_for_2_coils_linear_motion/Left_Coil/Inner 5 Coils/Coil-1 ==
  data: dxp_dz output; x_new input; y_new input; z_new input; dxn_dz output; dyp_dz output; dyn_dz output
function  [dxp_dz, dxn_dz, dyp_dz, dyn_dz] = current(x_new, y_new, z_new)

g = 520e-6;     %Coil spacing
m0 = 4*pi*1e-7;
radius = 3e-3;%m
height = 1e-3;%m
Magentization = 1.45; %T
vol_cy = pi*radius^2*height; % If Object is Cylinder, vol in m^3
% vol_sp = (4/3)*(pi * radius^3); % If Object is Sphere, vol in m^3

k = 0.4e-3; %additional length added to wires, to get concentric coil
%--------%--------%--------%--------%--------%--------%--------%----------
% Line along y - axis
%-%--------%--------%--------%--------%--------%--------%--------%--------
yp1_1 = -0.6e-3 ;
yp2_1 = 0.6e-3 ;
yn1_1 = -0.8e-3 ;
yn2_1 = 0.8e-3;
a_xp_1 = g;  
a_xn_1 = -g;

k_yp_1 = 1/(4*pi*((a_xp_1-x_new)^2+z_new^2));
k_1yp_1 = (yp2_1-y_new)/((yp2_1-y_new)^2+(a_xp_1-x_new)^2+z_new^2)^0.5;
k_2yp_1 = (yp1_1-y_new)/((yp1_1-y_new)^2+(a_xp_1-x_new)^2+z_new^2)^0.5;

k_1yp_3 = (yp2_1-y_new)/((yp2_1-y_new)^2+(a_xp_1-x_new)^2+z_new^2)^1.5;
k_2yp_3 = (yp1_1-y_new)/((yp1_1-y_new)^2+(a_xp_1-x_new)^2+z_new^2)^1.5;

k_yn_1 = 1/(4*pi*((a_xn_1-x_new)^2+z_new^2));
k_1yn_1 = (yn2_1-y_new)/((yn2_1-y_new)^2+(a_xn_1-x_new)^2+z_new^2)^0.5;
k_2yn_1 = (yn1_1-y_new)/((yn1_1-y_new)^2+(a_xn_1-x_new)^2+z_new^2)^0.5;

k_1yn_3 = (yn2_1-y_new)/((yn2_1-y_new)^2+(a_xn_1-x_new)^2+z_new^2)^1.5;
k_2yn_3 = (yn1_1-y_new)/((yn1_1-y_new)^2+(a_xn_1-x_new)^2+z_new^2)^1.5;


hyp_z_1 = (k_yp_1) *m0;
hyp_z1_1 = (k_1yp_1 - k_2yp_1)*(-1);
hyp_z2_1 = (k_yp_1*(k_1yp_1 - k_2yp_1)*(z_new^2))*4*pi*2;
hyp_z3_1 = (k_1yp_3 - k_2yp_3)*(z_new^2);
dxp_dz = hyp_z_1*(hyp_z1_1 + hyp_z2_1 + hyp_z3_1);


hyn_z_1 = (k_yn_1)* m0*(-1);
hyn_z1_1 = (k_1yn_1 - k_2yn_1)*(-1);
hyn_z2_1 = (k_yn_1*(k_1yn_1 - k_2yn_1)*(z_new^2))*4*pi*2;
hyn_z3_1 = (k_1yn_3 - k_2yn_3)*(z_new^2);
dxn_dz = hyn_z_1*(hyn_z1_1 + hyn_z2_1 + hyn_z3_1);

%--------%--------%--------%--------%--------%--------%--------%----------
% Line along x - axis
%-%--------%--------%--------%--------%a--------%--------%--------%--------
xp1_1 = -0.8e-3 ;
xp2_1 = 0.8e-3 ;
xn1_1 = -1e-3 ;
xn2_1 = 1e-3 ;
a_yp_1 = 0.675;          %Distance of coil from (0,0)
a_yn_1 = -0.675;

k_xp_1 = 1/(4*pi*((a_yp_1-y_new)^2+z_new^2));
k_1xp_1 = (xp2_1-x_new)/((xp2_1-x_new)^2+(a_yp_1-y_new)^2+z_new^2)^0.5;
k_2xp_1 = (xp1_1-x_new)/((xp1_1-x_new)^2+(a_yp_1-y_new)^2+z_new^2)^0.5;

k_xn_1 = 1/(4*pi*((a_yn_1-y_new)^2+z_new^2));
k_1xn_1 = (xn2_1-x_new)/((xn2_1-x_new)^2+(a_yn_1-y_new)^2+z_new^2)^0.5;
k_2xn_1 = (xn1_1-x_new)/((xn1_1-x_new)^2+(a_yn_1-y_new)^2+z_new^2)^0.5;

k_1xp_3 = (xp2_1-x_new)/((xp2_1-x_new)^2+(a_yp_1-y_new)^2+z_new^2)^1.5;
k_2xp_3 = (xp1_1-x_new)/((xp1_1-x_new)^2+(a_yp_1-y_new)^2+z_new^2)^1.5;

k_1xn_3 = (xn2_1-x_new)/((xn2_1-x_new)^2+(a_yn_1-y_new)^2+z_new^2)^1.5;
k_2xn_3 = (xn1_1-x_new)/((xn1_1-x_new)^2+(a_yn_1-y_new)^2+z_new^2)^1.5;


hxp_z_1 = (k_xp_1)*m0;
hxp_z1_1 = (k_1xp_1 - k_2xp_1)*(-1);
hxp_z2_1 = (k_xp_1*(k_1xp_1 - k_2xp_1)*(z_new^2))*4*pi*2;
hxp_z3_1 = (k_1xp_3 - k_2xp_3)*(z_new^2);
dyp_dz = hxp_z_1*(hxp_z1_1 + hxp_z2_1 + hxp_z3_1);


hxn_z_1 = (k_xn_1)*m0*(-1);
hxn_z1_1 = (k_1xn_1 - k_2xn_1)*(-1);
hxn_z2_1 = (k_xn_1*(k_1xn_1 - k_2xn_1)*(z_new^2))*4*pi*2;
hxn_z3_1 = (k_1xn_3 - k_2xn_3)*(z_new^2);
dyn_dz = hxn_z_1*(hxn_z1_1 + hxn_z2_1 + hxn_z3_1);

end

== matlab function I_for_2_coils_linear_motion/Left_Coil/Inner 5 Coils/Coil-2 ==
  data: dxp_dz output; x_new input; y_new input; z_new input; dxn_dz output; dyp_dz output; dyn_dz output
function  [dxp_dz, dxn_dz, dyp_dz, dyn_dz] = current(x_new, y_new, z_new)

g = 460e-6;     %Coil spacing
m0 = 4*pi*1e-7;
radius = 3e-3;%m
height = 1e-3;%m
Magentization = 1.45; %T
vol_cy = pi*radius^2*height; % If Object is Cylinder, vol in m^3
% vol_sp = (4/3)*(pi * radius^3); % If Object is Sphere, vol in m^3

k = 0.4e-3; %additional length added to wires, to get concentric coil
%--------%--------%--------%--------%--------%--------%--------%----------
% Line along y - axis
%-%--------%--------%--------%--------%--------%--------%--------%--------
yp1_1 = -0.6e-3 - k;
yp2_1 = 0.6e-3 + k;
yn1_1 = -0.8e-3 - k;
yn2_1 = 0.8e-3 + k;
a_xp_1 = 2*g;  
a_xn_1 = -2*g;

k_yp_1 = 1/(4*pi*((a_xp_1-x_new)^2+z_new^2));
k_1yp_1 = (yp2_1-y_new)/((yp2_1-y_new)^2+(a_xp_1-x_new)^2+z_new^2)^0.5;
k_2yp_1 = (yp1_1-y_new)/((yp1_1-y_new)^2+(a_xp_1-x_new)^2+z_new^2)^0.5;

k_1yp_3 = (yp2_1-y_new)/((yp2_1-y_new)^2+(a_xp_1-x_new)^2+z_new^2)^1.5;
k_2yp_3 = (yp1_1-y_new)/((yp1_1-y_new)^2+(a_xp_1-x_new)^2+z_new^2)^1.5;

k_yn_1 = 1/(4*pi*((a_xn_1-x_new)^2+z_new^2));
k_1yn_1 = (yn2_1-y_new)/((yn2_1-y_new)^2+(a_xn_1-x_new)^2+z_new^2)^0.5;
k_2yn_1 = (yn1_1-y_new)/((yn1_1-y_new)^2+(a_xn_1-x_new)^2+z_new^2)^0.5;

k_1yn_3 = (yn2_1-y_new)/((yn2_1-y_new)^2+(a_xn_1-x_new)^2+z_new^2)^1.5;
k_2yn_3 = (yn1_1-y_new)/((yn1_1-y_new)^2+(a_xn_1-x_new)^2+z_new^2)^1.5;


hyp_z_1 = (k_yp_1) *m0;
hyp_z1_1 = (k_1yp_1 - k_2yp_1)*(-1);
hyp_z2_1 = (k_yp_1*(k_1yp_1 - k_2yp_1)*(z_new^2))*4*pi*2;
hyp_z3_1 = (k_1yp_3 - k_2yp_3)*(z_new^2);
dxp_dz = hyp_z_1*(hyp_z1_1 + hyp_z2_1 + hyp_z3_1);


hyn_z_1 = (k_yn_1)* m0*(-1);
hyn_z1_1 = (k_1yn_1 - k_2yn_1)*(-1);
hyn_z2_1 = (k_yn_1*(k_1yn_1 - k_2yn_1)*(z_new^2))*4*pi*2;
hyn_z3_1 = (k_1yn_3 - k_2yn_3)*(z_new^2);
dxn_dz = hyn_z_1*(hyn_z1_1 + hyn_z2_1 + hyn_z3_1);

%--------%--------%--------%--------%--------%--------%--------%----------
% Line along x - axis
%-%--------%--------%--------%--------%a--------%--------%--------%--------
xp1_1 = -0.8e-3 - k;
xp2_1 = 0.8e-3 + k;
xn1_1 = -1e-3 - k;
xn2_1 = 1e-3 + k;
a_yp_1 = 1.075;          %Distance of coil from (0,0)
a_yn_1 = -1.075;

k_xp_1 = 1/(4*pi*((a_yp_1-y_new)^2+z_new^2));
k_1xp_1 = (xp2_1-x_new)/((xp2_1-x_new)^2+(a_yp_1-y_new)^2+z_new^2)^0.5;
k_2xp_1 = (xp1_1-x_new)/((xp1_1-x_new)^2+(a_yp_1-y_new)^2+z_new^2)^0.5;

k_xn_1 = 1/(4*pi*((a_yn_1-y_new)^2+z_new^2));
k_1xn_1 = (xn2_1-x_new)/((xn2_1-x_new)^2+(a_yn_1-y_new)^2+z_new^2)^0.5;
k_2xn_1 = (xn1_1-x_new)/((xn1_1-x_new)^2+(a_yn_1-y_new)^2+z_new^2)^0.5;

k_1xp_3 = (xp2_1-x_new)/((xp2_1-x_new)^2+(a_yp_1-y_new)^2+z_new^2)^1.5;
k_2xp_3 = (xp1_1-x_new)/((xp1_1-x_new)^2+(a_yp_1-y_new)^2+z_new^2)^1.5;

k_1xn_3 = (xn2_1-x_new)/((xn2_1-x_new)^2+(a_yn_1-y_new)^2+z_new^2)^1.5;
k_2xn_3 = (xn1_1-x_new)/((xn1_1-x_new)^2+(a_yn_1-y_new)^2+z_new^2)^1.5;


hxp_z_1 = (k_xp_1)*m0;
hxp_z1_1 = (k_1xp_1 - k_2xp_1)*(-1);
hxp_z2_1 = (k_xp_1*(k_1xp_1 - k_2xp_1)*(z_new^2))*4*pi*2;
hxp_z3_1 = (k_1xp_3 - k_2xp_3)*(z_new^2);
dyp_dz = hxp_z_1*(hxp_z1_1 + hxp_z2_1 + hxp_z3_1);


hxn_z_1 = (k_xn_1)*m0*(-1);
hxn_z1_1 = (k_1xn_1 - k_2xn_1)*(-1);
hxn_z2_1 = (k_xn_1*(k_1xn_1 - k_2xn_1)*(z_new^2))*4*pi*2;
hxn_z3_1 = (k_1xn_3 - k_2xn_3)*(z_new^2);
dyn_dz = hxn_z_1*(hxn_z1_1 + hxn_z2_1 + hxn_z3_1);

end

== matlab function I_for_2_coils_linear_motion/Left_Coil/Inner 5 Coils/Coil-3 ==
  data: dxp_dz output; x_new input; y_new input; z_new input; dxn_dz output; dyp_dz output; dyn_dz output
function  [dxp_dz, dxn_dz, dyp_dz, dyn_dz] = current(x_new, y_new, z_new)

g = 440e-6;     %Coil spacing
m0 = 4*pi*1e-7;
radius = 3e-3;%m
height = 1e-3;%m
Magentization = 1.45; %T
vol_cy = pi*radius^2*height; % If Object is Cylinder, vol in m^3
% vol_sp = (4/3)*(pi * radius^3); % If Object is Sphere, vol in m^3

k = 0.4e-3; %additional length added to wires, to get concentric coil
%--------%--------%--------%--------%--------%--------%--------%----------
% Line along y - axis
%-%--------%--------%--------%--------%--------%--------%--------%--------
yp1_1 = -0.6e-3 - 2*k;
yp2_1 = 0.6e-3 + 2*k;
yn1_1 = -0.8e-3 - 2*k;
yn2_1 = 0.8e-3 + 2*k;
a_xp_1 = 3*g;  
a_xn_1 = -3*g;

k_yp_1 = 1/(4*pi*((a_xp_1-x_new)^2+z_new^2));
k_1yp_1 = (yp2_1-y_new)/((yp2_1-y_new)^2+(a_xp_1-x_new)^2+z_new^2)^0.5;
k_2yp_1 = (yp1_1-y_new)/((yp1_1-y_new)^2+(a_xp_1-x_new)^2+z_new^2)^0.5;

k_1yp_3 = (yp2_1-y_new)/((yp2_1-y_new)^2+(a_xp_1-x_new)^2+z_new^2)^1.5;
k_2yp_3 = (yp1_1-y_new)/((yp1_1-y_new)^2+(a_xp_1-x_new)^2+z_new^2)^1.5;

k_yn_1 = 1/(4*pi*((a_xn_1-x_new)^2+z_new^2));
k_1yn_1 = (yn2_1-y_new)/((yn2_1-y_new)^2+(a_xn_1-x_new)^2+z_new^2)^0.5;
k_2yn_1 = (yn1_1-y_new)/((yn1_1-y_new)^2+(a_xn_1-x_new)^2+z_new^2)^0.5;

k_1yn_3 = (yn2_1-y_new)/((yn2_1-y_new)^2+(a_xn_1-x_new)^2+z_new^2)^1.5;
k_2yn_3 = (yn1_1-y_new)/((yn1_1-y_new)^2+(a_xn_1-x_new)^2+z_new^2)^1.5;


hyp_z_1 = (k_yp_1) *m0;
hyp_z1_1 = (k_1yp_1 - k_2yp_1)*(-1);
hyp_z2_1 = (k_yp_1*(k_1yp_1 - k_2yp_1)*(z_new^2))*4*pi*2;
hyp_z3_1 = (k_1yp_3 - k_2yp_3)*(z_new^2);
dxp_dz = hyp_z_1*(hyp_z1_1 + hyp_z2_1 + hyp_z3_1);


hyn_z_1 = (k_yn_1)* m0*(-1);
hyn_z1_1 = (k_1yn_1 - k_2yn_1)*(-1);
hyn_z2_1 = (k_yn_1*(k_1yn_1 - k_2yn_1)*(z_new^2))*4*pi*2;
hyn_z3_1 = (k_1yn_3 - k_2yn_3)*(z_new^2);
dxn_dz = hyn_z_1*(hyn_z1_1 + hyn_z2_1 + hyn_z3_1);

%--------%--------%--------%--------%--------%--------%--------%----------
% Line along x - axis
%-%--------%--------%--------%--------%a--------%--------%--------%--------
xp1_1 = -0.8e-3 - 2*k;
xp2_1 = 0.8e-3 + 2*k;
xn1_1 = -1e-3 - 2*k;
xn2_1 = 1e-3 + 2*k;
a_yp_1 = 1.475;          %Distance of coil from (0,0)
a_yn_1 = -1.475;

k_xp_1 = 1/(4*pi*((a_yp_1-y_new)^2+z_new^2));
k_1xp_1 = (xp2_1-x_new)/((xp2_1-x_new)^2+(a_yp_1-y_new)^2+z_new^2)^0.5;
k_2xp_1 = (xp1_1-x_new)/((xp1_1-x_new)^2+(a_yp_1-y_new)^2+z_new^2)^0.5;

k_xn_1 = 1/(4*pi*((a_yn_1-y_new)^2+z_new^2));
k_1xn_1 = (xn2_1-x_new)/((xn2_1-x_new)^2+(a_yn_1-y_new)^2+z_new^2)^0.5;
k_2xn_1 = (xn1_1-x_new)/((xn1_1-x_new)^2+(a_yn_1-y_new)^2+z_new^2)^0.5;

k_1xp_3 = (xp2_1-x_new)/((xp2_1-x_new)^2+(a_yp_1-y_new)^2+z_new^2)^1.5;
k_2xp_3 = (xp1_1-x_new)/((xp1_1-x_new)^2+(a_yp_1-y_new)^2+z_new^2)^1.5;

k_1xn_3 = (xn2_1-x_new)/((xn2_1-x_new)^2+(a_yn_1-y_new)^2+z_new^2)^1.5;
k_2xn_3 = (xn1_1-x_new)/((xn1_1-x_new)^2+(a_yn_1-y_new)^2+z_new^2)^1.5;


hxp_z_1 = (k_xp_1)*m0;
hxp_z1_1 = (k_1xp_1 - k_2xp_1)*(-1);
hxp_z2_1 = (k_xp_1*(k_1xp_1 - k_2xp_1)*(z_new^2))*4*pi*2;
hxp_z3_1 = (k_1xp_3 - k_2xp_3)*(z_new^2);
dyp_dz = hxp_z_1*(hxp_z1_1 + hxp_z2_1 + hxp_z3_1);


hxn_z_1 = (k_xn_1)*m0*(-1);
hxn_z1_1 = (k_1xn_1 - k_2xn_1)*(-1);
hxn_z2_1 = (k_xn_1*(k_1xn_1 - k_2xn_1)*(z_new^2))*4*pi*2;
hxn_z3_1 = (k_1xn_3 - k_2xn_3)*(z_new^2);
dyn_dz = hxn_z_1*(hxn_z1_1 + hxn_z2_1 + hxn_z3_1);

end

== matlab function I_for_2_coils_linear_motion/Left_Coil/Inner 5 Coils/Coil-4 ==
  data: dxp_dz output; x_new input; y_new input; z_new input; dxn_dz output; dyp_dz output; dyn_dz output
function  [dxp_dz, dxn_dz, dyp_dz, dyn_dz] = current(x_new, y_new, z_new)

g = 430e-6;     %Coil spacing
m0 = 4*pi*1e-7;
radius = 3e-3;%m
height = 1e-3;%m
Magentization = 1.45; %T
vol_cy = pi*radius^2*height; % If Object is Cylinder, vol in m^3
% vol_sp = (4/3)*(pi * radius^3); % If Object is Sphere, vol in m^3

k = 0.4e-3; %additional length added to wires, to get concentric coil
%--------%--------%--------%--------%--------%--------%--------%----------
% Line along y - axis
%-%--------%--------%--------%--------%--------%--------%--------%--------
yp1_1 = -0.6e-3 - 3*k;
yp2_1 = 0.6e-3 + 3*k;
yn1_1 = -0.8e-3 - 3*k;
yn2_1 = 0.8e-3 + 3*k;
a_xp_1 = 4*g;  
a_xn_1 = -4*g;

k_yp_1 = 1/(4*pi*((a_xp_1-x_new)^2+z_new^2));
k_1yp_1 = (yp2_1-y_new)/((yp2_1-y_new)^2+(a_xp_1-x_new)^2+z_new^2)^0.5;
k_2yp_1 = (yp1_1-y_new)/((yp1_1-y_new)^2+(a_xp_1-x_new)^2+z_new^2)^0.5;

k_1yp_3 = (yp2_1-y_new)/((yp2_1-y_new)^2+(a_xp_1-x_new)^2+z_new^2)^1.5;
k_2yp_3 = (yp1_1-y_new)/((yp1_1-y_new)^2+(a_xp_1-x_new)^2+z_new^2)^1.5;

k_yn_1 = 1/(4*pi*((a_xn_1-x_new)^2+z_new^2));
k_1yn_1 = (yn2_1-y_new)/((yn2_1-y_new)^2+(a_xn_1-x_new)^2+z_new^2)^0.5;
k_2yn_1 = (yn1_1-y_new)/((yn1_1-y_new)^2+(a_xn_1-x_new)^2+z_new^2)^0.5;

k_1yn_3 = (yn2_1-y_new)/((yn2_1-y_new)^2+(a_xn_1-x_new)^2+z_new^2)^1.5;
k_2yn_3 = (yn1_1-y_new)/((yn1_1-y_new)^2+(a_xn_1-x_new)^2+z_new^2)^1.5;


hyp_z_1 = (k_yp_1) *m0;
hyp_z1_1 = (k_1yp_1 - k_2yp_1)*(-1);
hyp_z2_1 = (k_yp_1*(k_1yp_1 - k_2yp_1)*(z_new^2))*4*pi*2;
hyp_z3_1 = (k_1yp_3 - k_2yp_3)*(z_new^2);
dxp_dz = hyp_z_1*(hyp_z1_1 + hyp_z2_1 + hyp_z3_1);


hyn_z_1 = (k_yn_1)* m0*(-1);
hyn_z1_1 = (k_1yn_1 - k_2yn_1)*(-1);
hyn_z2_1 = (k_yn_1*(k_1yn_1 - k_2yn_1)*(z_new^2))*4*pi*2;
hyn_z3_1 = (k_1yn_3 - k_2yn_3)*(z_new^2);
dxn_dz = hyn_z_1*(hyn_z1_1 + hyn_z2_1 + hyn_z3_1);

%--------%--------%--------%--------%--------%--------%--------%----------
% Line along x - axis
%-%--------%--------%--------%--------%a--------%--------%--------%--------
xp1_1 = -0.8e-3 - 3*k;
xp2_1 = 0.8e-3 + 3*k;
xn1_1 = -1e-3 - 3*k;
xn2_1 = 1e-3 + 3*k;
a_yp_1 = 1.875;          %Distance of coil from (0,0)
a_yn_1 = -1.875;

k_xp_1 = 1/(4*pi*((a_yp_1-y_new)^2+z_new^2));
k_1xp_1 = (xp2_1-x_new)/((xp2_1-x_new)^2+(a_yp_1-y_new)^2+z_new^2)^0.5;
k_2xp_1 = (xp1_1-x_new)/((xp1_1-x_new)^2+(a_yp_1-y_new)^2+z_new^2)^0.5;

k_xn_1 = 1/(4*pi*((a_yn_1-y_new)^2+z_new^2));
k_1xn_1 = (xn2_1-x_new)/((xn2_1-x_new)^2+(a_yn_1-y_new)^2+z_new^2)^0.5;
k_2xn_1 = (xn1_1-x_new)/((xn1_1-x_new)^2+(a_yn_1-y_new)^2+z_new^2)^0.5;

k_1xp_3 = (xp2_1-x_new)/((xp2_1-x_new)^2+(a_yp_1-y_new)^2+z_new^2)^1.5;
k_2xp_3 = (xp1_1-x_new)/((xp1_1-x_new)^2+(a_yp_1-y_new)^2+z_new^2)^1.5;

k_1xn_3 = (xn2_1-x_new)/((xn2_1-x_new)^2+(a_yn_1-y_new)^2+z_new^2)^1.5;
k_2xn_3 = (xn1_1-x_new)/((xn1_1-x_new)^2+(a_yn_1-y_new)^2+z_new^2)^1.5;


hxp_z_1 = (k_xp_1)*m0;
hxp_z1_1 = (k_1xp_1 - k_2xp_1)*(-1);
hxp_z2_1 = (k_xp_1*(k_1xp_1 - k_2xp_1)*(z_new^2))*4*pi*2;
hxp_z3_1 = (k_1xp_3 - k_2xp_3)*(z_new^2);
dyp_dz = hxp_z_1*(hxp_z1_1 + hxp_z2_1 + hxp_z3_1);


hxn_z_1 = (k_xn_1)*m0*(-1);
hxn_z1_1 = (k_1xn_1 - k_2xn_1)*(-1);
hxn_z2_1 = (k_xn_1*(k_1xn_1 - k_2xn_1)*(z_new^2))*4*pi*2;
hxn_z3_1 = (k_1xn_3 - k_2xn_3)*(z_new^2);
dyn_dz = hxn_z_1*(hxn_z1_1 + hxn_z2_1 + hxn_z3_1);

end

== matlab function I_for_2_coils_linear_motion/Left_Coil/Inner 5 Coils/Coil-5 ==
  data: dxp_dz output; x_new input; y_new input; z_new input; dxn_dz output; dyp_dz output; dyn_dz output
function  [dxp_dz, dxn_dz, dyp_dz, dyn_dz] = current(x_new, y_new, z_new)

g = 424e-6;     %Coil spacing
m0 = 4*pi*1e-7;
radius = 3e-3;%m
height = 1e-3;%m
Magentization = 1.45; %T
vol_cy = pi*radius^2*height; % If Object is Cylinder, vol in m^3
% vol_sp = (4/3)*(pi * radius^3); % If Object is Sphere, vol in m^3

k = 0.4e-3; %additional length added to wires, to get concentric coil
%--------%--------%--------%--------%--------%--------%--------%----------
% Line along y - axis
%-%--------%--------%--------%--------%--------%--------%--------%--------
yp1_1 = -0.6e-3 - 4*k;
yp2_1 = 0.6e-3 + 4*k;
yn1_1 = -0.8e-3 - 4*k;
yn2_1 = 0.8e-3 + 4*k;
a_xp_1 = 5*g;  
a_xn_1 = -5*g;

k_yp_1 = 1/(4*pi*((a_xp_1-x_new)^2+z_new^2));
k_1yp_1 = (yp2_1-y_new)/((yp2_1-y_new)^2+(a_xp_1-x_new)^2+z_new^2)^0.5;
k_2yp_1 = (yp1_1-y_new)/((yp1_1-y_new)^2+(a_xp_1-x_new)^2+z_new^2)^0.5;

k_1yp_3 = (yp2_1-y_new)/((yp2_1-y_new)^2+(a_xp_1-x_new)^2+z_new^2)^1.5;
k_2yp_3 = (yp1_1-y_new)/((yp1_1-y_new)^2+(a_xp_1-x_new)^2+z_new^2)^1.5;

k_yn_1 = 1/(4*pi*((a_xn_1-x_new)^2+z_new^2));
k_1yn_1 = (yn2_1-y_new)/((yn2_1-y_new)^2+(a_xn_1-x_new)^2+z_new^2)^0.5;
k_2yn_1 = (yn1_1-y_new)/((yn1_1-y_new)^2+(a_xn_1-x_new)^2+z_new^2)^0.5;

k_1yn_3 = (yn2_1-y_new)/((yn2_1-y_new)^2+(a_xn_1-x_new)^2+z_new^2)^1.5;
k_2yn_3 = (yn1_1-y_new)/((yn1_1-y_new)^2+(a_xn_1-x_new)^2+z_new^2)^1.5;


hyp_z_1 = (k_yp_1) *m0;
hyp_z1_1 = (k_1yp_1 - k_2yp_1)*(-1);
hyp_z2_1 = (k_yp_1*(k_1yp_1 - k_2yp_1)*(z_new^2))*4*pi*2;
hyp_z3_1 = (k_1yp_3 - k_2yp_3)*(z_new^2);
dxp_dz = hyp_z_1*(hyp_z1_1 + hyp_z2_1 + hyp_z3_1);


hyn_z_1 = (k_yn_1)* m0*(-1);
hyn_z1_1 = (k_1yn_1 - k_2yn_1)*(-1);
hyn_z2_1 = (k_yn_1*(k_1yn_1 - k_2yn_1)*(z_new^2))*4*pi*2;
hyn_z3_1 = (k_1yn_3 - k_2yn_3)*(z_new^2);
dxn_dz = hyn_z_1*(hyn_z1_1 + hyn_z2_1 + hyn_z3_1);

%--------%--------%--------%--------%--------%--------%--------%----------
% Line along x - axis
%-%--------%--------%--------%--------%a--------%--------%--------%--------
xp1_1 = -0.8e-3 - 4*k;
xp2_1 = 0.8e-3 + 4*k;
xn1_1 = -1e-3 - 4*k;
xn2_1 = 1e-3 + 4*k;
a_yp_1 = 2.275;          %Distance of coil from (0,0)
a_yn_1 = -2.275;

k_xp_1 = 1/(4*pi*((a_yp_1-y_new)^2+z_new^2));
k_1xp_1 = (xp2_1-x_new)/((xp2_1-x_new)^2+(a_yp_1-y_new)^2+z_new^2)^0.5;
k_2xp_1 = (xp1_1-x_new)/((xp1_1-x_new)^2+(a_yp_1-y_new)^2+z_new^2)^0.5;

k_xn_1 = 1/(4*pi*((a_yn_1-y_new)^2+z_new^2));
k_1xn_1 = (xn2_1-x_new)/((xn2_1-x_new)^2+(a_yn_1-y_new)^2+z_new^2)^0.5;
k_2xn_1 = (xn1_1-x_new)/((xn1_1-x_new)^2+(a_yn_1-y_new)^2+z_new^2)^0.5;

k_1xp_3 = (xp2_1-x_new)/((xp2_1-x_new)^2+(a_yp_1-y_new)^2+z_new^2)^1.5;
k_2xp_3 = (xp1_1-x_new)/((xp1_1-x_new)^2+(a_yp_1-y_new)^2+z_new^2)^1.5;

k_1xn_3 = (xn2_1-x_new)/((xn2_1-x_new)^2+(a_yn_1-y_new)^2+z_new^2)^1.5;
k_2xn_3 = (xn1_1-x_new)/((xn1_1-x_new)^2+(a_yn_1-y_new)^2+z_new^2)^1.5;


hxp_z_1 = (k_xp_1)*m0;
hxp_z1_1 = (k_1xp_1 - k_2xp_1)*(-1);
hxp_z2_1 = (k_xp_1*(k_1xp_1 - k_2xp_1)*(z_new^2))*4*pi*2;
hxp_z3_1 = (k_1xp_3 - k_2xp_3)*(z_new^2);
dyp_dz = hxp_z_1*(hxp_z1_1 + hxp_z2_1 + hxp_z3_1);


hxn_z_1 = (k_xn_1)*m0*(-1);
hxn_z1_1 = (k_1xn_1 - k_2xn_1)*(-1);
hxn_z2_1 = (k_xn_1*(k_1xn_1 - k_2xn_1)*(z_new^2))*4*pi*2;
hxn_z3_1 = (k_1xn_3 - k_2xn_3)*(z_new^2);
dyn_dz = hxn_z_1*(hxn_z1_1 + hxn_z2_1 + hxn_z3_1);

end
